simulink model "blance_leg"  (R2023b)
settings: Solver=VariableStepAuto  StartTime=0.0  StopTime=10  MaxStep=0.24  RelTol=1e-3
undefined symbols (not defined in the file or in its folder): k11, k110, k12, k13, k14, k15, k16, k17, k18, k19, k21, k210, k22, k23, k24, k25, k26, k27, k28, k29, k31, k310, k32, k33, k34, k35, k36, k37, k38, k39, k41, k410, k42, k43, k44, k45, k46, k47, k48, k49, X, Y, Z
libraries: sm_lib x114, nesl_utility x23, matrix_library x4, slpidlib x2
(part 1 of 4)
settings Model: SimulationMode=accelerator  Creator=Hhop  LastModifiedBy=erink
settings SolverCC: ZeroCrossAlgorithm=Adaptive  MinimalZcImpactIntegration=on
settings OptimizationCC: ReuseModelBlockBuffer=off
settings DebuggingCC: ReadBeforeWriteMsg=DisableAll  WriteAfterWriteMsg=DisableAll  WriteAfterReadMsg=DisableAll  IgnoredZcDiagnostic=none  MultiTaskDSMMsg=none
settings ModelReferenceCC: UpdateModelReferenceTargets=IfOutOfDate
settings SFSimCC: SFSimEcho=off

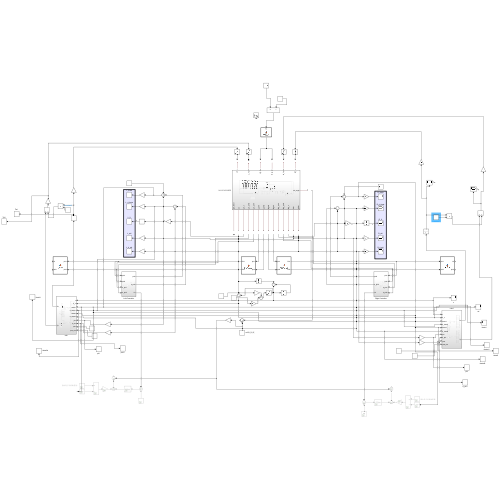
[thumbnail: Simulink's stored preview of the top-level diagram]
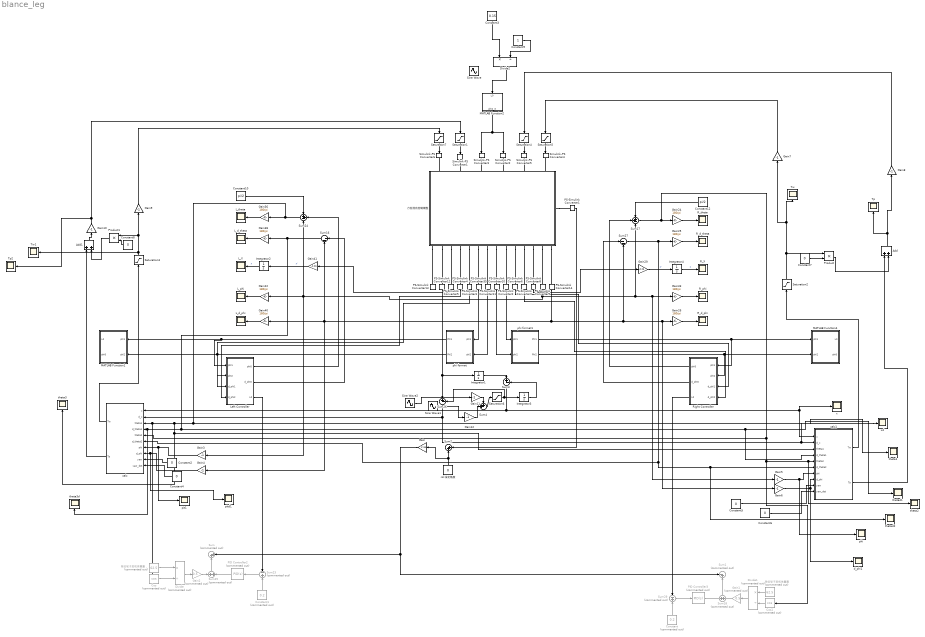
== system blance_leg ==
  Add : Sum
  Add1 : Sum
  Constant : Constant  Commented=on  Value=0.2
  Constant1 : Constant  Commented=on  Value=0.2
  Constant10 : Constant  Value=pi/2
  Constant12 : Constant  Value=pi/2
  Constant{2,4..8} (6 alike) : Constant  Value=0
  Constant3 : Constant  Value=0.15
  Constant9 : Constant
  Cos : Trigonometry  Commented=on  Operator=cos
  Cos1 : Trigonometry  Commented=on  Operator=cos
  Divide : Product  Commented=on  Inputs=*/
  Divide1 : Product  Commented=on  Inputs=*/
  Divide2 : Product  Inputs=*/
  Gain : Gain  Gain=1700
  Gain1 : Gain  Commented=on  Gain=0.5
  Gain{3..12} (10 alike) : Gain  Gain=-1
  Gain2 : Gain  Commented=on  Gain=0.5
  Gain{22,24..26,33,36,38,40} (8 alike) : Gain  Gain=180/pi
  Gain29 : Gain  Gain=-0.06
  Gain41 : Gain  Gain=-0.06
  Integrator{1..4} (4 alike) : Integrator
  L_X : Scope
  L_d_phi : Scope
  L_d_theta : Scope
  L_phi : Scope
  L_theta : Scope
  Left Controller : Subsystem
  MATLAB Function1 : MATLAB Function  TreatAsAtomicUnit=on
  MATLAB Function2 : MATLAB Function  TreatAsAtomicUnit=on
  MATLAB Function4 : MATLAB Function  TreatAsAtomicUnit=on
  PID Controller2 : slpidlib/PID Controller  Commented=on  Controller=PID  Form=Parallel  TimeDomain=Continuous-time  UseExternalTs=off  SampleTime=-1  IntegratorMethod=Forward Euler  FilterMethod=Forward Euler  ControllerParametersSource=internal  P=500  I=0  UseKiTs=off  D=200  N=100  UseFilter=on  TunerSelectOption=Transfer Function Based (PID Tuner App)  InitialConditionSource=internal  InitialConditionForIntegrator=0  InitialConditionForFilter=0  DifferentiatorICPrevScaledInput=0  ExternalReset=none  TrackingMode=off  Kt=1  LimitOutput=off  SatLimitsSource=internal  UpperSaturationLimit=inf  LowerSaturationLimit=-inf  LinearizeAsGain=on  AntiWindupMode=none  Kb=1  LimitIntegrator=off  UpperIntegratorSaturationLimit=inf  LowerIntegratorSaturationLimit=-inf  POutMin=[]  POutMax=[]  IOutMin=[]  IOutMax=[]  DOutMin=[]  DOutMax=[]  NOutMin=[]  NOutMax=[]  SumOutMin=[]  SumOutMax=[]  SaturationOutMin=[]  SaturationOutMax=[]  PParamMin=[]  PParamMax=[]  IParamMin=[]  IParamMax=[]  DParamMin=[]  DParamMax=[]  NParamMin=[]  NParamMax=[]  KbParamMin=[]  KbParamMax=[]  KtParamMin=[]  KtParamMax=[]  KbOutMin=[]  KbOutMax=[]  KtOutMin=[]  KtOutMax=[]  IntegratorOutMin=[]  IntegratorOutMax=[]  FilterOutMin=[]  FilterOutMax=[]  SumI1OutMin=[]  SumI1OutMax=[]  SumI2OutMin=[]  SumI2OutMax=[]  SumI3OutMin=[]  SumI3OutMax=[]  SumI4OutMin=[]  SumI4OutMax=[]  SumDOutMin=[]  SumDOutMax=[]  DifferentiatorOutMin=[]  DifferentiatorOutMax=[]  FilterDiffOutCoefMin=[]  FilterDiffOutCoefMax=[]  ReciprocalOutMin=[]  ReciprocalOutMax=[]  SumDenOutMin=[]  SumDenOutMax=[]  SumNumOutMin=[]  SumNumOutMax=[]  DivideOutMin=[]  DivideOutMax=[]  UdiffTsProdOutMin=[]  UdiffTsProdOutMax=[]  NTsProdOutMin=[]  NTsProdOutMax=[]  UintegralTsProdOutMin=[]  UintegralTsProdOutMax=[]  UngainTsProdOutMin=[]  UngainTsProdOutMax=[]  ClampingZeroOutDataTypeStr=Inherit: Inherit via back propagation  ClampingZeroOutMin=[]  ClampingZeroOutMax=[]  FilterDenConstantOutDataTypeStr=Inherit: Inherit via back propagation  FilterDenConstantOutMin=[]  FilterDenConstantOutMax=[]  PCopyOutDataTypeStr=Inherit: Inherit via back propagation  PCopyOutMin=[]  PCopyOutMax=[]  NCopyOutDataTypeStr=Inherit: Inherit via back propagation  NCopyOutMin=[]  NCopyOutMax=[]  IntegratorContinuousStateAttributes=''  IntegratorStateMustResolveToSignalObject=off  IntegratorRTWStateStorageClass=Auto  FilterContinuousStateAttributes=''  FilterStateMustResolveToSignalObject=off  FilterRTWStateStorageClass=Auto  ParallelPVariant=InternalParameters  IdealPVariant=Disabled  IVariant=InternalParameters  DVariant=InternalParameters  IntegratorVariant=Continuous  SatVariant=Disabled  AWVariant=Passthrough  PCopyVariant=Disabled  TRVariant=Disabled  FdbkBlocksVariant=Forward  IdealPFdbkVariant=Disabled  SatFdbkVariant=Disabled  DerivativeFilterVariant=ContFilter  NVariant=InternalParameters  NCopyVariant=Disabled  FilterICVariant=InternalICsFilter  IntegratorICVariant=InternalICs  ExternalResetVariant=Disabled  TRSumVariant=Passthrough  SumFdbkVariant=Disabled  SumVariant=Sum_PID  TsampFilterVariant=InternalTs  TsampNgainVariant=Passthrough  TsampIntegralVariant=Disabled_SignalSpec  ExternalSaturationOutDataTypeStr=Inherit: Same as second input
  PID Controller3 : slpidlib/PID Controller  Commented=on  Controller=PID  Form=Parallel  TimeDomain=Continuous-time  UseExternalTs=off  SampleTime=-1  IntegratorMethod=Forward Euler  FilterMethod=Forward Euler  ControllerParametersSource=internal  P=500  I=0  UseKiTs=off  D=200  N=100  UseFilter=on  TunerSelectOption=Transfer Function Based (PID Tuner App)  InitialConditionSource=internal  InitialConditionForIntegrator=0  InitialConditionForFilter=0  DifferentiatorICPrevScaledInput=0  ExternalReset=none  TrackingMode=off  Kt=1  LimitOutput=off  SatLimitsSource=internal  UpperSaturationLimit=inf  LowerSaturationLimit=-inf  LinearizeAsGain=on  AntiWindupMode=none  Kb=1  LimitIntegrator=off  UpperIntegratorSaturationLimit=inf  LowerIntegratorSaturationLimit=-inf  POutMin=[]  POutMax=[]  IOutMin=[]  IOutMax=[]  DOutMin=[]  DOutMax=[]  NOutMin=[]  NOutMax=[]  SumOutMin=[]  SumOutMax=[]  SaturationOutMin=[]  SaturationOutMax=[]  PParamMin=[]  PParamMax=[]  IParamMin=[]  IParamMax=[]  DParamMin=[]  DParamMax=[]  NParamMin=[]  NParamMax=[]  KbParamMin=[]  KbParamMax=[]  KtParamMin=[]  KtParamMax=[]  KbOutMin=[]  KbOutMax=[]  KtOutMin=[]  KtOutMax=[]  IntegratorOutMin=[]  IntegratorOutMax=[]  FilterOutMin=[]  FilterOutMax=[]  SumI1OutMin=[]  SumI1OutMax=[]  SumI2OutMin=[]  SumI2OutMax=[]  SumI3OutMin=[]  SumI3OutMax=[]  SumI4OutMin=[]  SumI4OutMax=[]  SumDOutMin=[]  SumDOutMax=[]  DifferentiatorOutMin=[]  DifferentiatorOutMax=[]  FilterDiffOutCoefMin=[]  FilterDiffOutCoefMax=[]  ReciprocalOutMin=[]  ReciprocalOutMax=[]  SumDenOutMin=[]  SumDenOutMax=[]  SumNumOutMin=[]  SumNumOutMax=[]  DivideOutMin=[]  DivideOutMax=[]  UdiffTsProdOutMin=[]  UdiffTsProdOutMax=[]  NTsProdOutMin=[]  NTsProdOutMax=[]  UintegralTsProdOutMin=[]  UintegralTsProdOutMax=[]  UngainTsProdOutMin=[]  UngainTsProdOutMax=[]  ClampingZeroOutDataTypeStr=Inherit: Inherit via back propagation  ClampingZeroOutMin=[]  ClampingZeroOutMax=[]  FilterDenConstantOutDataTypeStr=Inherit: Inherit via back propagation  FilterDenConstantOutMin=[]  FilterDenConstantOutMax=[]  PCopyOutDataTypeStr=Inherit: Inherit via back propagation  PCopyOutMin=[]  PCopyOutMax=[]  NCopyOutDataTypeStr=Inherit: Inherit via back propagation  NCopyOutMin=[]  NCopyOutMax=[]  IntegratorContinuousStateAttributes=''  IntegratorStateMustResolveToSignalObject=off  IntegratorRTWStateStorageClass=Auto  FilterContinuousStateAttributes=''  FilterStateMustResolveToSignalObject=off  FilterRTWStateStorageClass=Auto  ParallelPVariant=InternalParameters  IdealPVariant=Disabled  IVariant=InternalParameters  DVariant=InternalParameters  IntegratorVariant=Continuous  SatVariant=Disabled  AWVariant=Passthrough  PCopyVariant=Disabled  TRVariant=Disabled  FdbkBlocksVariant=Forward  IdealPFdbkVariant=Disabled  SatFdbkVariant=Disabled  DerivativeFilterVariant=ContFilter  NVariant=InternalParameters  NCopyVariant=Disabled  FilterICVariant=InternalICsFilter  IntegratorICVariant=InternalICs  ExternalResetVariant=Disabled  TRSumVariant=Passthrough  SumFdbkVariant=Disabled  SumVariant=Sum_PID  TsampFilterVariant=InternalTs  TsampNgainVariant=Passthrough  TsampIntegralVariant=Disabled_SignalSpec  ExternalSaturationOutDataTypeStr=Inherit: Same as second input
  PS-Simulink Converter{1..14,35} (15 alike) : nesl_utility/PS-Simulink Converter  PhysicalDomain=network_engine_domain  SubClassName=ps_output  LeftPortType=input  RightPortType=output  PseudoPeriodic=off  Frequencies=[]  VectorFormat=inherit  Unit=inherit  AffineConversion=off
  Product : Product
  Product1 : Product
  R_X : Scope
  R_d_phi : Scope
  R_d_theta : Scope
  R_phi : Scope
  R_theta : Scope
  Right Controller : Subsystem
  Saturation{1,4..5,7} (4 alike) : Saturate  UpperLimit=20  LowerLimit=-20
  Saturation2 : Saturate  UpperLimit=5  LowerLimit=-5
  Saturation3 : Saturate  UpperLimit=5  LowerLimit=-5
  Saturation6 : Saturate  UpperLimit=4  LowerLimit=-4
  Simulink-PS Converter{1,4..6} (4 alike) : nesl_utility/Simulink-PS Converter  PhysicalDomain=network_engine_domain  SubClassName=ps_input  LeftPortType=input  RightPortType=output  PseudoPeriodic=off  Frequencies=[]  NoiseDistribution=none  NoiseParameters=[]  Unit=1  AffineConversion=off  FilteringAndDerivatives=provide  SimscapeFilterOrder=1  InputFilterTimeConstant=0.001  UdotUserProvided=0
  Simulink-PS Converter2 : nesl_utility/Simulink-PS Converter  PhysicalDomain=network_engine_domain  SubClassName=ps_input  LeftPortType=input  RightPortType=output  PseudoPeriodic=off  Frequencies=[]  NoiseDistribution=none  NoiseParameters=[]  Unit=1  AffineConversion=off  FilteringAndDerivatives=filter  SimscapeFilterOrder=2  InputFilterTimeConstant=0.001  UdotUserProvided=0
  Simulink-PS Converter3 : nesl_utility/Simulink-PS Converter  PhysicalDomain=network_engine_domain  SubClassName=ps_input  LeftPortType=input  RightPortType=output  PseudoPeriodic=off  Frequencies=[]  NoiseDistribution=none  NoiseParameters=[]  Unit=1  AffineConversion=off  FilteringAndDerivatives=filter  SimscapeFilterOrder=2  InputFilterTimeConstant=0.001  UdotUserProvided=0
  Sine Wave : Sin  Amplitude=0.01  Bias=0.18  Frequency=2  SampleTime=0
  Sine Wave1 : Sin  Frequency=2  Phase=2  SampleTime=0
  Sine Wave2 : Sin  Frequency=2  Phase=1  SampleTime=0
  Sum : Sum  Commented=on  Inputs=|++
  Sum1 : Sum  Commented=on  Inputs=-+|
  Sum16 : Sum  Inputs=|--
  Sum17 : Sum  Inputs=+--
  Sum18 : Sum  Commented=on  Inputs=+|+
  Sum2 : Sum  Inputs=|++
  Sum23 : Sum  Commented=on  Inputs=-|+
  Sum24 : Sum  Inputs=+--
  Sum25 : Sum  Commented=on  Inputs=+|+
  Sum26 : Sum  Inputs=|+-
  Sum27 : Sum  Inputs=|--
  Sum29 : Sum  Commented=on  Inputs=-|+
  Sum3 : Sum  Inputs=|+-
  Sum4 : Sum  Inputs=++|
  Tp : Scope
  Tp2 : Scope
  Tw : Scope
  Tw1 : Scope
  calc : Subsystem
  calc1 : Subsystem
  d_phi1 : Scope
  phi : Scope
  phi format : MATLAB Function  TreatAsAtomicUnit=on
  phi format1 : MATLAB Function  TreatAsAtomicUnit=on
  pit1 : Scope
  pitd1 : Scope
  roll设定角度 : Constant  Value=0
  theta1 : Scope
  theta2 : Scope
  theta3 : Scope
  theta3d : Scope
  thetad1 : Scope
  thetad2 : Scope
  x : Scope
  xd : Scope
  力位混合控制模型 : Subsystem
      settings: PortSchema="{\"entries\":[{\"content\":{\"sides\":[{\"content\":{\"connectorIds\":[\"LConn1\",\"LConn2\",\"LConn3\",\"LConn4\",\"LConn5\",\"LConn6\"]},\"type\":\"ConnectorPlacement.EquallySpacedRectSide\",\"uuid\":\"ed635f35-0836-4900-93e3-56fc3520c8de\"},{\"content\":{\"connectorIds\":[\"RConn1\",\"RConn2\",\"RConn3\",\"RConn4\",\"RConn5\",\"RConn6\",\"RConn7\",\"RConn8\",\"RConn9\",\"RConn10\",\"RConn11\",\"RConn12\",\"RConn13\",\"RConn14\"],\"side\":\"RIGHT\"},\"type\":\"ConnectorPlacement.EquallySpacedRectSide\",\"uuid\":\"bb235ec0-defd-4ad9-96f6-8533dab3fbd9\"},{\"content\":{\"side\":\"TOP\"},\"type\":\"ConnectorPlacement.EquallySpacedRectSide\",\"uuid\":\"d719db37-8b3a-4344-b330-944fde418334\"},{\"content\":{\"connectorIds\":[\"RConn15\"],\"side\":\"BOTTOM\"},\"type\":\"ConnectorPlacement.EquallySpacedRectSide\",\"uuid\":\"20f9270b-6ab1-4e89-bf00-e838d12c3c13\"}]},\"type\":\"ConnectorPlacement.EquallySpacedConnector\",\"uuid\":\"a2f25b71-0047-4a2d-a238-dad76f034ab1\"}],\"packageUris\":[\"http://schema.mathworks.com/mf0/Connector/R2020b\"],\"version\":\"1.0\"}"
  除去轮子后机体重量 : Constant  Commented=on  Value=62.5
  除去轮子后机体重量， : Constant  Commented=on  Value=62.5
  wires:
  Constant12/1 -> Sum17/1
  Gain40/1 -> L_d_phi/1
  Constant/1 -> Sum29/2
  Sum23/1 -> PID Controller2/1
  Right Controller/1(phi0) -> Sum17/2
  Gain33/1 -> R_phi/1
  Right Controller/3(L0) -> Sum29/1
  PID Controller3/1 -> Sum18/1
  Integrator4/1 -> R_X/1  "x"
  PID Controller2/1 -> Sum25/2
  Gain22/1 -> L_phi/1
  Constant10/1 -> Sum24/1
  Integrator2/1 -> L_X/1  "x"
  Sum29/1 -> PID Controller3/1
  Gain26/1 -> R_d_phi/1
  Gain24/1 -> R_theta/1
  Sum25/1 -> Sum/1
  Sum18/1 -> Sum1/2
  Gain38/1 -> L_d_theta/1
  Right Controller/2(d_phi0) -> Sum27/1
  Gain41/1 -> Integrator2/1  "x'"
  Constant1/1 -> Sum23/2
  Gain36/1 -> L_theta/1
  Gain25/1 -> R_d_theta/1
  Gain29/1 -> Integrator4/1  "x'"
  除去轮子后机体重量，/1 -> Divide/1
  Cos/1 -> Divide/2
  Cos1/1 -> Divide1/2
  除去轮子后机体重量/1 -> Divide1/1
  PS-Simulink Converter35/1 -> phi format/1(phi1)
  PS-Simulink Converter11/1 -> phi format/2(phi2)
  PS-Simulink Converter2/1 -> phi format1/1(phi1)
  PS-Simulink Converter10/1 -> phi format1/2(phi2)
  phi format1/1(Phi1) -> Right Controller/1(phi1), MATLAB Function4/1(phi1)
  phi format1/2(Phi2) -> Right Controller/2(phi2), MATLAB Function4/2(phi2)
  PS-Simulink Converter8/1 -> Gain29/1
  PS-Simulink Converter6/1 -> Right Controller/3(d_phi1)
  PS-Simulink Converter7/1 -> Right Controller/4(d_phi2)
  phi format/1(Phi1) -> Left Controller/4(phi1), MATLAB Function1/1(phi1)
  phi format/2(Phi2) -> Left Controller/3(phi2), MATLAB Function1/2(phi2)
  PS-Simulink Converter3/1 -> Left Controller/2(d_phi1)
  PS-Simulink Converter4/1 -> Left Controller/1(d_phi2)
  PS-Simulink Converter5/1 -> Gain41/1
  PS-Simulink Converter9/1 -> Gain22/1, Gain3/1, Sum24/3, Sum17/3, Gain5/1, Gain33/1
  PS-Simulink Converter14/1 -> Gain40/1, Gain4/1, Sum16/2, Sum27/2, Gain6/1, Gain26/1
  Left Controller/2(d_phi0) -> Sum16/1
  Left Controller/3(phi0) -> Sum24/2
  Left Controller/1(L0) -> Sum23/1
  PS-Simulink Converter12/1 -> Integrator1/1, Sum26/1
  PS-Simulink Converter1/1 -> Sum2/1
  roll设定角度/1 -> Gain/1, Sum2/2
  Gain/1 -> Sum1/1, Sum/2
  Saturation7/1 -> Simulink-PS Converter6/1
  Saturation1/1 -> Simulink-PS Converter1/1
  Saturation4/1 -> Simulink-PS Converter5/1
  Saturation5/1 -> Simulink-PS Converter4/1
  Divide1/1 -> Gain1/1
  Divide/1 -> Gain2/1
  Gain1/1 -> Sum18/2
  Gain2/1 -> Sum25/1
  MATLAB Function2/1(phi2_3) -> Simulink-PS Converter3/1, Simulink-PS Converter2/1
  Saturation6/1 -> Sum26/2, Integrator3/1
  Sine Wave2/1 -> Gain11/1
  Integrator1/1 -> Sum3/1
  Integrator3/1 -> Sum3/2
  Gain3/1 -> pit1/1, calc/7(phi)
  Gain4/1 -> pitd1/1, calc/8(d_phi)
  Gain5/1 -> phi/1, calc1/7(phi)
  Gain6/1 -> calc1/8(d_phi), d_phi1/1
  Constant2/1 -> calc/9(yaw)
  Constant4/1 -> calc/10(yaw_dot)
  Constant5/1 -> calc1/9(yaw)
  Constant6/1 -> calc1/10(yaw_dot)
  calc1/1(Tw) -> Saturation2/1
  calc/1(Tw) -> Saturation3/1
  Sum3/1 -> calc/1(x), calc1/1(x), x/1
  Sum26/1 -> calc/2(d_x), xd/1, calc1/2(d_x)
  Saturation2/1 -> Gain7/1, Tw/1, Product/1
  Saturation3/1 -> Gain9/1, Product1/1, Tw1/1
  Gain7/1 -> Saturation5/1
  Gain8/1 -> Saturation4/1
  Sum24/1 -> calc/3(theta1), Cos/1, calc1/3(theta1), theta3/1, theta1/1, Gain36/1
  Sum16/1 -> calc1/4(d_theta1), thetad1/1, theta3d/1, calc/4(d_theta1), Gain38/1
  Sum17/1 -> calc/5(theta2), Cos1/1, theta2/1, calc1/5(theta2), Gain24/1
  Sum27/1 -> calc/6(d_theta2), calc1/6(d_theta2), thetad2/1, Gain25/1
  Gain9/1 -> Saturation7/1
  Gain10/1 -> Tp2/1, Saturation1/1
  Gain11/1 -> Sum4/1
  Sum4/1 -> Saturation6/1
  Sine Wave1/1 -> Gain12/1
  Gain12/1 -> Sum4/2
  Constant3/1 -> Divide2/1
  Constant9/1 -> Divide2/2
  Divide2/1 -> MATLAB Function2/1(L0)
  Constant7/1 -> Product/2
  Product/1 -> Add/2
  calc1/2(Tp) -> Add/1
  Add/1 -> Tp/1, Gain8/1
  Constant8/1 -> Product1/2
  calc/2(Tp) -> Add1/1
  Product1/1 -> Add1/2
  Add1/1 -> Gain10/1
  connections:
  力位混合控制模型/LConn3 -- Simulink-PS Converter3/RConn1
  力位混合控制模型/LConn2 -- Simulink-PS Converter1/RConn1
  力位混合控制模型/RConn15 -- PS-Simulink Converter1/LConn1
  力位混合控制模型/LConn4 -- Simulink-PS Converter2/RConn1
  力位混合控制模型/LConn5 -- Simulink-PS Converter5/RConn1
  力位混合控制模型/LConn1 -- Simulink-PS Converter6/RConn1
  力位混合控制模型/LConn6 -- Simulink-PS Converter4/RConn1
  力位混合控制模型/RConn2 -- PS-Simulink Converter12/LConn1
  力位混合控制模型/RConn6 -- PS-Simulink Converter35/LConn1
  力位混合控制模型/RConn1 -- PS-Simulink Converter13/LConn1
  力位混合控制模型/RConn9 -- PS-Simulink Converter2/LConn1
  力位混合控制模型/RConn14 -- PS-Simulink Converter14/LConn1
  力位混合控制模型/RConn10 -- PS-Simulink Converter6/LConn1
  力位混合控制模型/RConn4 -- PS-Simulink Converter4/LConn1
  力位混合控制模型/RConn8 -- PS-Simulink Converter10/LConn1
  力位混合控制模型/RConn13 -- PS-Simulink Converter9/LConn1
  力位混合控制模型/RConn12 -- PS-Simulink Converter8/LConn1
  力位混合控制模型/RConn5 -- PS-Simulink Converter3/LConn1
  力位混合控制模型/RConn11 -- PS-Simulink Converter7/LConn1
  力位混合控制模型/RConn7 -- PS-Simulink Converter11/LConn1
  力位混合控制模型/RConn3 -- PS-Simulink Converter5/LConn1

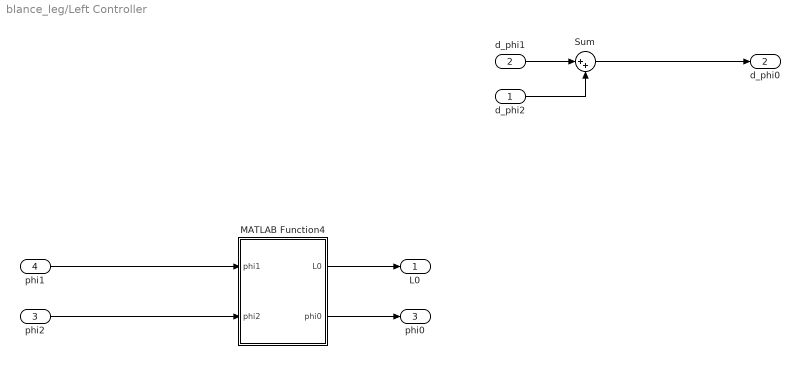
== system blance_leg/Left Controller ==
  d_phi2 : Inport
  d_phi1 : Inport  Port=2
  phi2 : Inport  Port=3
  phi1 : Inport  Port=4
  MATLAB Function4 : MATLAB Function  TreatAsAtomicUnit=on
  Sum : Sum  Inputs=|++
  L0 : Outport
  d_phi0 : Outport  Port=2
  phi0 : Outport  Port=3
  wires:
  phi1/1 -> MATLAB Function4/1(phi1)
  d_phi1/1 -> Sum/1
  d_phi2/1 -> Sum/2
  MATLAB Function4/1(L0) -> L0/1
  MATLAB Function4/2(phi0) -> phi0/1
  phi2/1 -> MATLAB Function4/2(phi2)
  Sum/1 -> d_phi0/1

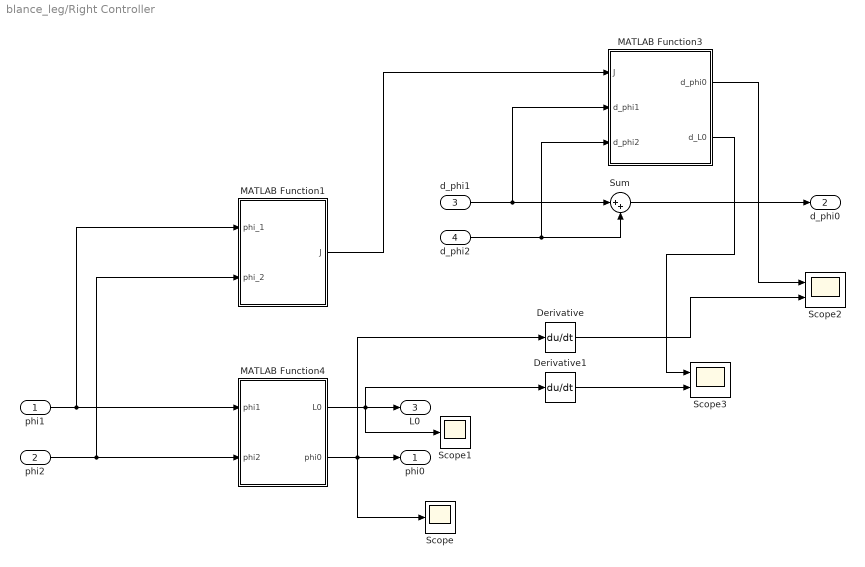
== system blance_leg/Right Controller ==
  phi1 : Inport
  phi2 : Inport  Port=2
  d_phi1 : Inport  Port=3
  d_phi2 : Inport  Port=4
  Derivative : Derivative
  Derivative1 : Derivative
  MATLAB Function1 : MATLAB Function  TreatAsAtomicUnit=on
  MATLAB Function3 : MATLAB Function  TreatAsAtomicUnit=on
  MATLAB Function4 : MATLAB Function  TreatAsAtomicUnit=on
  Scope : Scope
  Scope1 : Scope
  Scope2 : Scope  NumInputPorts=2
  Scope3 : Scope  NumInputPorts=2
  Sum : Sum  Inputs=|++
  phi0 : Outport
  d_phi0 : Outport  Port=2
  L0 : Outport  Port=3
  wires:
  phi1/1 -> MATLAB Function1/1(phi_1), MATLAB Function4/1(phi1)
  MATLAB Function4/2(phi0) -> Derivative/1, Scope/1, phi0/1
  phi2/1 -> MATLAB Function1/2(phi_2), MATLAB Function4/2(phi2)
  MATLAB Function4/1(L0) -> Derivative1/1, Scope1/1, L0/1
  Derivative/1 -> Scope2/2
  d_phi1/1 -> MATLAB Function3/2(d_phi1), Sum/1
  MATLAB Function1/1(J) -> MATLAB Function3/1(J)
  MATLAB Function3/1(d_phi0) -> Scope2/1
  d_phi2/1 -> MATLAB Function3/3(d_phi2), Sum/2
  Sum/1 -> d_phi0/1
  Derivative1/1 -> Scope3/2
  MATLAB Function3/2(d_L0) -> Scope3/1

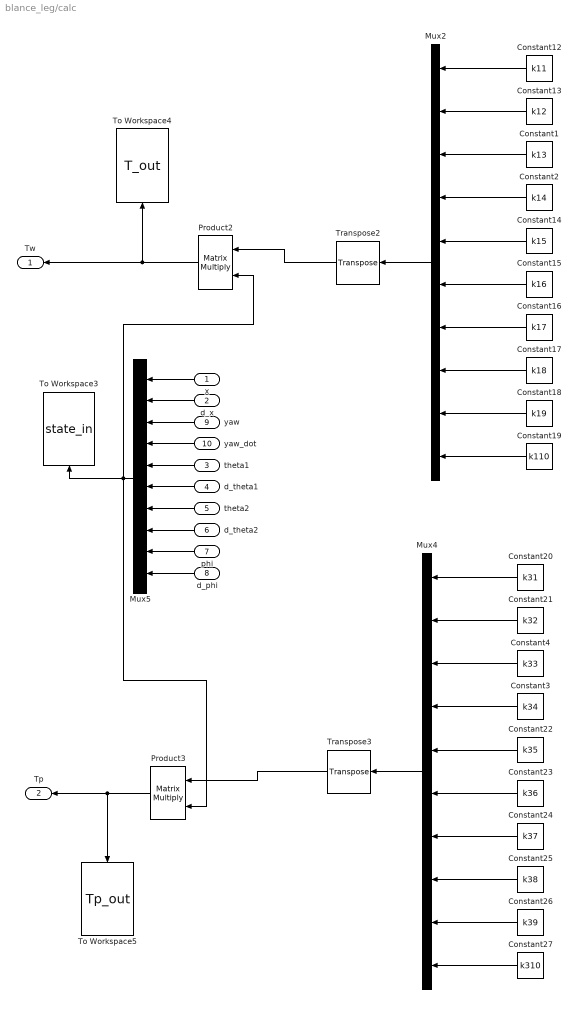
== system blance_leg/calc ==
  x : Inport
  d_x : Inport  Port=2
  theta1 : Inport  Port=3
  d_theta1 : Inport  Port=4
  theta2 : Inport  Port=5
  d_theta2 : Inport  Port=6
  phi : Inport  Port=7
  d_phi : Inport  Port=8
  yaw : Inport  Port=9
  yaw_dot : Inport  Port=10
  Constant1 : Constant  Value=k13
  Constant12 : Constant  Value=k11
  Constant13 : Constant  Value=k12
  Constant14 : Constant  Value=k15
  Constant15 : Constant  Value=k16
  Constant16 : Constant  Value=k17
  Constant17 : Constant  Value=k18
  Constant18 : Constant  Value=k19
  Constant19 : Constant  Value=k110
  Constant2 : Constant  Value=k14
  Constant20 : Constant  Value=k31
  Constant21 : Constant  Value=k32
  Constant22 : Constant  Value=k35
  Constant23 : Constant  Value=k36
  Constant24 : Constant  Value=k37
  Constant25 : Constant  Value=k38
  Constant26 : Constant  Value=k39
  Constant27 : Constant  Value=k310
  Constant3 : Constant  Value=k34
  Constant4 : Constant  Value=k33
  Mux2 : Mux  Inputs=10
  Mux4 : Mux  Inputs=10
  Mux5 : Mux  Inputs=10
  Product2 : Product  Multiplication=Matrix(*)
  Product3 : Product  Multiplication=Matrix(*)
  To Workspace3 : ToWorkspace  VariableName=state_in  SampleTime=-1
      settings: Save2DSignal=2-D array (concatenate along first dimension)
  To Workspace4 : ToWorkspace  VariableName=T_out  SampleTime=-1
      settings: Save2DSignal=2-D array (concatenate along first dimension)
  To Workspace5 : ToWorkspace  VariableName=Tp_out  SampleTime=-1
      settings: Save2DSignal=2-D array (concatenate along first dimension)
  Transpose2 : matrix_library/Transpose
  Transpose3 : matrix_library/Transpose
  Tw : Outport
  Tp : Outport  Port=2
  wires:
  Constant12/1 -> Mux2/1
  Constant13/1 -> Mux2/2
  Mux2/1 -> Transpose2/1
  Mux4/1 -> Transpose3/1
  Constant21/1 -> Mux4/2
  Constant20/1 -> Mux4/1
  x/1 -> Mux5/1
  d_x/1 -> Mux5/2
  phi/1 -> Mux5/9
  d_phi/1 -> Mux5/10
  theta1/1 -> Mux5/5
  d_theta1/1 -> Mux5/6
  theta2/1 -> Mux5/7
  d_theta2/1 -> Mux5/8
  yaw/1 -> Mux5/3
  yaw_dot/1 -> Mux5/4
  Mux5/1 -> To Workspace3/1, Product2/2, Product3/2
  Transpose2/1 -> Product2/1
  Transpose3/1 -> Product3/1
  Product2/1 -> Tw/1, To Workspace4/1
  Product3/1 -> Tp/1, To Workspace5/1
  Constant19/1 -> Mux2/10
  Constant18/1 -> Mux2/9
  Constant17/1 -> Mux2/8
  Constant16/1 -> Mux2/7
  Constant15/1 -> Mux2/6
  Constant14/1 -> Mux2/5
  Constant2/1 -> Mux2/4
  Constant1/1 -> Mux2/3
  Constant4/1 -> Mux4/3
  Constant3/1 -> Mux4/4
  Constant22/1 -> Mux4/5
  Constant23/1 -> Mux4/6
  Constant24/1 -> Mux4/7
  Constant25/1 -> Mux4/8
  Constant26/1 -> Mux4/9
  Constant27/1 -> Mux4/10

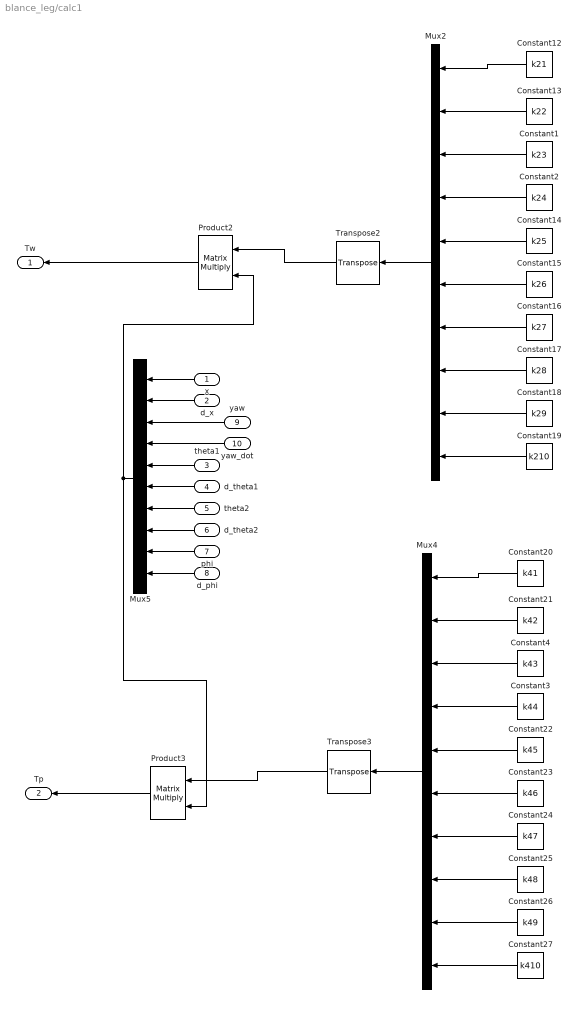
== system blance_leg/calc1 ==
  x : Inport
  d_x : Inport  Port=2
  theta1 : Inport  Port=3
  d_theta1 : Inport  Port=4
  theta2 : Inport  Port=5
  d_theta2 : Inport  Port=6
  phi : Inport  Port=7
  d_phi : Inport  Port=8
  yaw : Inport  Port=9
  yaw_dot : Inport  Port=10
  Constant1 : Constant  Value=k23
  Constant12 : Constant  Value=k21
  Constant13 : Constant  Value=k22
  Constant14 : Constant  Value=k25
  Constant15 : Constant  Value=k26
  Constant16 : Constant  Value=k27
  Constant17 : Constant  Value=k28
  Constant18 : Constant  Value=k29
  Constant19 : Constant  Value=k210
  Constant2 : Constant  Value=k24
  Constant20 : Constant  Value=k41
  Constant21 : Constant  Value=k42
  Constant22 : Constant  Value=k45
  Constant23 : Constant  Value=k46
  Constant24 : Constant  Value=k47
  Constant25 : Constant  Value=k48
  Constant26 : Constant  Value=k49
  Constant27 : Constant  Value=k410
  Constant3 : Constant  Value=k44
  Constant4 : Constant  Value=k43
  Mux2 : Mux  Inputs=10
  Mux4 : Mux  Inputs=10
  Mux5 : Mux  Inputs=10
  Product2 : Product  Multiplication=Matrix(*)
  Product3 : Product  Multiplication=Matrix(*)
  Transpose2 : matrix_library/Transpose
  Transpose3 : matrix_library/Transpose
  Tw : Outport
  Tp : Outport  Port=2
  wires:
  Constant12/1 -> Mux2/1
  Constant13/1 -> Mux2/2
  Mux2/1 -> Transpose2/1
  Mux4/1 -> Transpose3/1
  Constant21/1 -> Mux4/2
  Constant20/1 -> Mux4/1
  x/1 -> Mux5/1
  d_x/1 -> Mux5/2
  phi/1 -> Mux5/9
  d_phi/1 -> Mux5/10
  theta1/1 -> Mux5/5
  d_theta1/1 -> Mux5/6
  theta2/1 -> Mux5/7
  d_theta2/1 -> Mux5/8
  yaw/1 -> Mux5/3
  yaw_dot/1 -> Mux5/4
  Mux5/1 -> Product2/2, Product3/2
  Transpose2/1 -> Product2/1
  Transpose3/1 -> Product3/1
  Product2/1 -> Tw/1
  Product3/1 -> Tp/1
  Constant19/1 -> Mux2/10
  Constant18/1 -> Mux2/9
  Constant17/1 -> Mux2/8
  Constant16/1 -> Mux2/7
  Constant15/1 -> Mux2/6
  Constant14/1 -> Mux2/5
  Constant1/1 -> Mux2/3
  Constant2/1 -> Mux2/4
  Constant27/1 -> Mux4/10
  Constant26/1 -> Mux4/9
  Constant25/1 -> Mux4/8
  Constant24/1 -> Mux4/7
  Constant23/1 -> Mux4/6
  Constant22/1 -> Mux4/5
  Constant4/1 -> Mux4/3
  Constant3/1 -> Mux4/4
